simulink model "PMSM_FOC_MPC"  (R2024b)
settings: Solver=ode4  StartTime=0.0  StopTime=2  FixedStep=1e-6  RelTol=1e-3
InitFcn:
  | %% Motor Parameters
  | Rs = 0.9585;
  | Ls = 0.00525;
  | 
  | %% Observer Parameters
  | K = [817.42 0;
  |       0      817.42];
  | 
  | %% State Matrix
  | A = [ -Rs/Ls      0;
  |         0     -Rs/Ls ];
  | 
  | %% Input Matrix
  | B = [ 1/Ls      0;
  |         0     1/Ls ];
  | 
  | %% Output Matrix
  | C = [1 0;
  |      0 1];
  | 
  | %% Feedthrough
  | D = zeros(2,2);
values from neighbouring files (symbols this model uses):
  V = VPH - mean(VPH)    [three_level_inverter.m]
libraries: spsabctoAlphaBetaZeroLib x3, spsDCVoltageSourceLib x1, spsPermanentMagnetSynchronousMachineLib x1, spsThreePhaseVIMeasurementLib x1, spsUniversalBridgeLib x1, sps_lib x1, slpidlib x1
settings Model: SimulationMode=accelerator  Creator=killa  LastModifiedBy=killa

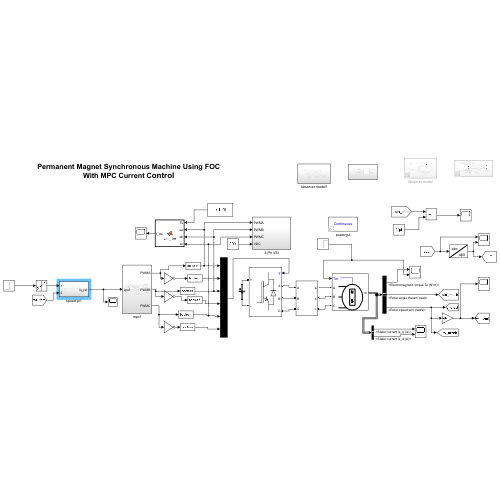
[thumbnail: Simulink's stored preview of the top-level diagram]
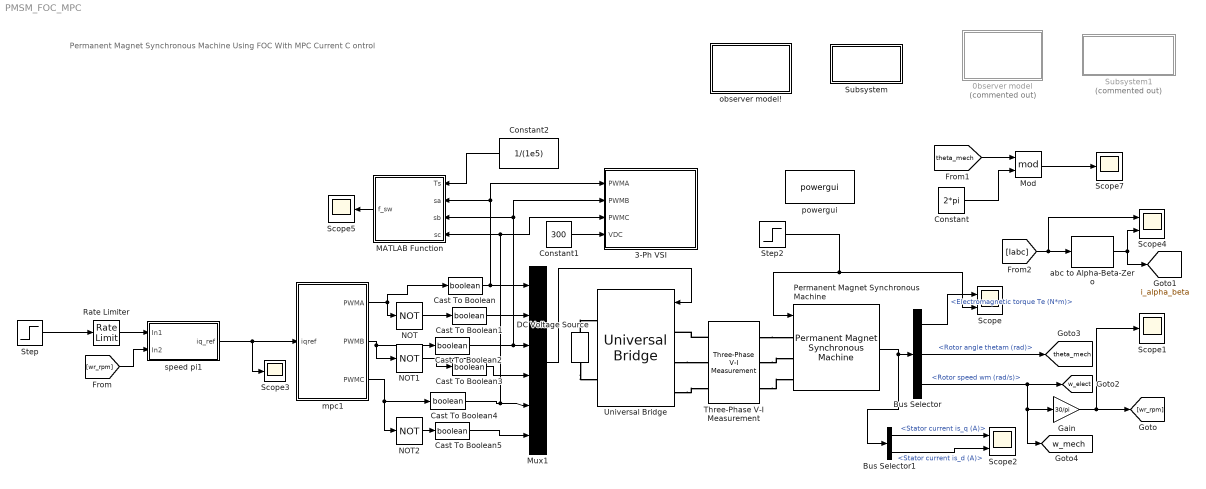
== system PMSM_FOC_MPC ==
  note: Permanent Magnet Synchronous Machine Using FOC With MPC Current C ontrol
  0bserver model : Subsystem  Commented=on
  3-Ph VSI : Subsystem
  Bus Selector : BusSelector  OutputSignals=Electromagnetic torque Te (N*m),Rotor angle thetam (rad),Rotor speed wm (rad/s)
  Bus Selector1 : BusSelector  OutputSignals=Stator current is_q (A),Stator current is_d (A)
  Cast To Boolean{,1..5} (6 alike) : DataTypeConversion  OutDataTypeStr=boolean  SaturateOnIntegerOverflow=off  RndMeth=Floor
  Constant : Constant  Value=2*pi
  Constant1 : Constant  Value=300
  Constant2 : Constant  Value=1/(1e5)
  DC Voltage Source : spsDCVoltageSourceLib/DC Voltage Source  Amplitude=300  Measurements=None
  Gain : Gain  Gain=30/pi
  MATLAB Function : MATLAB Function  TreatAsAtomicUnit=on
  Mod : Math  Operator=mod
  Mux1 : Mux  Inputs=6
  NOT : Logic  Operator=NOT  IconShape=distinctive  AllPortsSameDT=off  OutDataTypeStr=boolean
  NOT1 : Logic  Operator=NOT  IconShape=distinctive  AllPortsSameDT=off  OutDataTypeStr=boolean
  NOT2 : Logic  Operator=NOT  IconShape=distinctive  AllPortsSameDT=off  OutDataTypeStr=boolean
  Permanent Magnet Synchronous Machine : spsPermanentMagnetSynchronousMachineLib/Permanent Magnet Synchronous Machine  NbPhases=3  FluxDistribution=Sinusoidal  RotorType=Round  MechanicalLoad=Torque Tm  PresetModel="05:  8 Nm 300 Vdc 2000 RPM - 10 Nm"  ShowDetailedParameters=on  MeasurementBus=off  Resistance=0.9585  Inductance=8.5e-3  dqInductances=[8.5e-3,8.5e-3]  La=0.00525  MachineConstant=Flux linkage established by magnets (V.s)  Flux=0.1827  VoltageCst=132.5525  TorqueCst=1.0962  Flat=120  Mechanical=[0.0006329 0.0003035 4 0]  PolePairs=4  InitialConditions=[0,0, 0,0]  InitialConditions5ph=[0 0 0 0 0 0]  RefAngle=Aligned with phase A axis (original Park)  IterativeDiscreteModel=Trapezoidal non iterative  TsBlock=-1  TsPowergui=0
  Rate Limiter : RateLimiter  RisingSlewLimit=10000  FallingSlewLimit=-10000
  Scope : Scope  NumInputPorts=2
  Scope{1,3,5,7} (4 alike) : Scope
  Scope2 : Scope  NumInputPorts=2
  Scope4 : Scope  NumInputPorts=2
  Step : Step  Before=500  After=1500  SampleTime=0
  Step2 : Step  Time=0.5  Before=4  After=8  SampleTime=0
  Subsystem : Subsystem
  Subsystem1 : Subsystem  Commented=on
  Three-Phase V-I Measurement : spsThreePhaseVIMeasurementLib/Three-Phase V-I Measurement  VoltageMeasurement=no  SetLabelV=on  LabelV=Vabc  Vpu=off  VpuLL=off  CurrentMeasurement=yes  SetLabelI=on  LabelI=Iabc  Ipu=off  Pbase=100e6  Vbase=500e3  OutputType=Complex  PhasorSimulation=off  PSBequivalent=0
  Universal Bridge : spsUniversalBridgeLib/Universal Bridge  Arms=3  SnubberResistance=1e5  SnubberCapacitance=inf  Device=IGBT / Diodes  Ron=1e-3  Lon=0  ForwardVoltages="[  0  0  ]"  ForwardVoltage=0  GTOparameters=[ 10e-6 , 20e-6 ]  IGBTparameters=[ 1e-6 , 2e-6 ]  Measurements=None  Measurements_2=None  converterType=Rectifier
  abc to Alpha-Beta-Zero : spsabctoAlphaBetaZeroLib/abc to Alpha-Beta-Zero
  mpc1 : Subsystem
  observer model! : Subsystem
  powergui : sps_lib/powergui  Priority=1  SimulationMode=Continuous  SampleTime=50e-6  frequency=60  Iterations=50  frequencyindice=0  Pbase=100e6  ErrMax=1e-4  UnitsV=kV  UnitsW=MW  buscounter=0  FunctionMessages=off  echomessages=off  EnableUseOfTLC=off  CurrentSourceSwitches=off  DisableSnubberDevices=off  DisableRonSwitches=off  DisableVfSwitches=off  DisplayEquations=off  AutomaticDiscreteSolvers=off  SolverType=Tustin/Backward Euler (TBE)  Interpol=off  ExternalGateDelay=off  methode=off  Ts=100  x0status=blocks  SPID=on  SwTol=0  HookPort=off  NonlinearTolerance=1e-4  nMaxIteration=100  ContinueOnMaxIteration=off  RestoreLinks=warning  ResistiveCurrentMeasurement=off  Frange=[0:2:500]  Ylog=off  Xlog=on  ShowGrid=off  save=off  variable=ZData  structure=0  ZoomFFT=off  StartTime=0.0  cycles=1  DisplayStyle=1  fundamental=60  FreqAxis=off  MaxFrequency=1000  frequencyindicesteady=1  RmsSteady=1  display=off
  speed pi1 : Subsystem
  tag scope: i_alpha_beta=global, theta_mech=global, w_elect=global, w_mech=global
  wires:
  Permanent Magnet Synchronous Machine/1 -> Bus Selector1/1, Bus Selector/1
  Bus Selector/2 -> [theta_mech]  "<Rotor angle thetam (rad)>"
  Bus Selector/3 -> [w_mech], Gain/1, [w_elect]  "<Rotor speed wm (rad/s)>"
  Bus Selector/1 -> Scope/1  "<Electromagnetic torque Te (N*m)>"
  Gain/1 -> [wr_rpm], Scope1/1
  Cast To Boolean/1 -> Mux1/1, 3-Ph VSI/1(PWMA), MATLAB Function/2(sa)
  mpc1/1(PWMA) -> Cast To Boolean/1, NOT/1
  NOT/1 -> Cast To Boolean1/1
  Cast To Boolean1/1 -> Mux1/2
  mpc1/2(PWMB) -> Cast To Boolean2/1, NOT1/1
  NOT1/1 -> Cast To Boolean3/1
  mpc1/3(PWMC) -> Cast To Boolean4/1, NOT2/1
  NOT2/1 -> Cast To Boolean5/1
  Cast To Boolean2/1 -> 3-Ph VSI/2(PWMB), MATLAB Function/3(sb), Mux1/3
  Cast To Boolean3/1 -> Mux1/4
  Cast To Boolean4/1 -> 3-Ph VSI/3(PWMC), MATLAB Function/4(sc), Mux1/5
  Cast To Boolean5/1 -> Mux1/6
  Mux1/1 -> Universal Bridge/1
  [Iabc] -> abc to Alpha-Beta-Zero/1, Scope4/1
  Constant1/1 -> 3-Ph VSI/4(VDC)
  Step2/1 -> Scope/2, Permanent Magnet Synchronous Machine/1
  Bus Selector1/1 -> Scope2/1  "<Stator current is_q (A)>"
  Bus Selector1/2 -> Scope2/2  "<Stator current is_d (A)>"
  Constant2/1 -> MATLAB Function/1(Ts)
  MATLAB Function/1(f_sw) -> Scope5/1
  [wr_rpm] -> speed pi1/2(In2)
  speed pi1/1(iq_ref) -> mpc1/1(iqref), Scope3/1
  Step/1 -> Rate Limiter/1
  abc to Alpha-Beta-Zero/1 -> [i_alpha_beta], Scope4/2
  [theta_mech] -> Mod/1
  Constant/1 -> Mod/2
  Mod/1 -> Scope7/1
  Rate Limiter/1 -> speed pi1/1(In1)
  connections:
  DC Voltage Source/RConn1 -- Universal Bridge/RConn1
  DC Voltage Source/LConn1 -- Universal Bridge/RConn2
  Three-Phase V-I Measurement/LConn1 -- Universal Bridge/LConn1
  Universal Bridge/LConn2 -- Three-Phase V-I Measurement/LConn2
  Universal Bridge/LConn3 -- Three-Phase V-I Measurement/LConn3
  Three-Phase V-I Measurement/RConn1 -- Permanent Magnet Synchronous Machine/LConn1
  Three-Phase V-I Measurement/RConn2 -- Permanent Magnet Synchronous Machine/LConn2
  Three-Phase V-I Measurement/RConn3 -- Permanent Magnet Synchronous Machine/LConn3

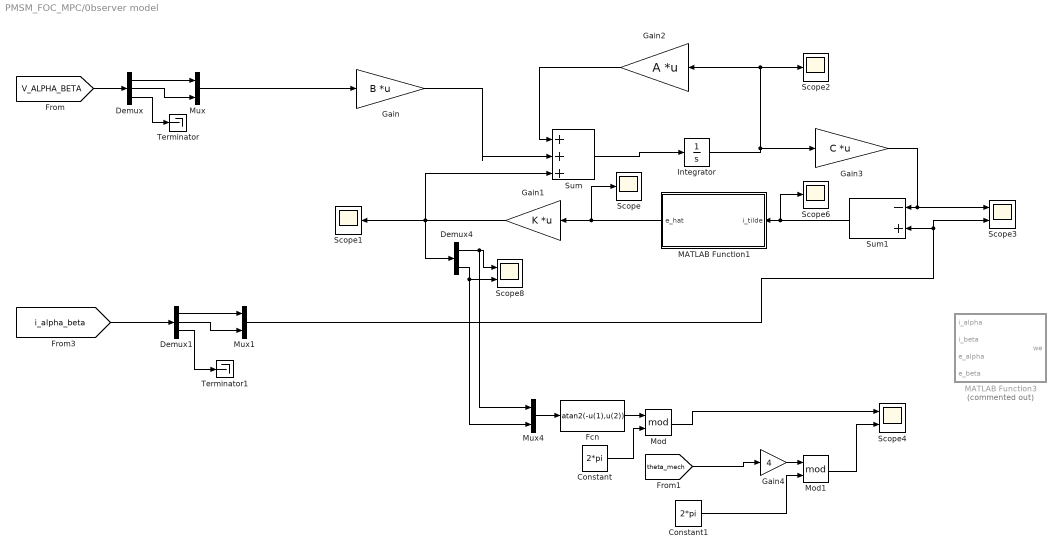
== system PMSM_FOC_MPC/0bserver model ==
  Constant : Constant  Value=2*pi
  Constant1 : Constant  Value=2*pi
  Demux : Demux  Outputs=3
  Demux1 : Demux  Outputs=3
  Demux4 : Demux  Outputs=2
  Fcn : Fcn  Expr=atan2(-u(1),u(2))
  Gain : Gain  Gain=B  Multiplication=Matrix(K*u)
  Gain1 : Gain  Gain=K  Multiplication=Matrix(K*u)
  Gain2 : Gain  Gain=A  Multiplication=Matrix(K*u)
  Gain3 : Gain  Gain=C  Multiplication=Matrix(K*u)
  Gain4 : Gain  Gain=4
  Integrator : Integrator
  MATLAB Function1 : MATLAB Function  TreatAsAtomicUnit=on
  MATLAB Function3 : MATLAB Function  Commented=on  TreatAsAtomicUnit=on
  Mod : Math  Operator=mod
  Mod1 : Math  Operator=mod
  Mux : Mux  Inputs=2
  Mux1 : Mux  Inputs=2
  Mux4 : Mux  Inputs=2
  Scope{,1..2,6} (4 alike) : Scope
  Scope3 : Scope  NumInputPorts=2
  Scope4 : Scope  NumInputPorts=2
  Scope8 : Scope  NumInputPorts=2
  Sum : Sum  Inputs=|+++
  Sum1 : Sum  Inputs=-+
  Terminator : Terminator
  Terminator1 : Terminator
  wires:
  Integrator/1 -> Scope2/1, Gain2/1, Gain3/1
  Gain2/1 -> Sum/1
  Fcn/1 -> Mod/1
  Sum/1 -> Integrator/1
  Constant/1 -> Mod/2
  Gain/1 -> Sum/2
  Mux4/1 -> Fcn/1
  Gain3/1 -> Scope3/1, Sum1/1
  [V_ALPHA_BETA] -> Demux/1
  Demux/1 -> Mux/1
  Demux/2 -> Mux/2
  Mux/1 -> Gain/1
  Demux/3 -> Terminator/1
  Demux1/1 -> Mux1/1
  Demux1/2 -> Mux1/2
  Demux1/3 -> Terminator1/1
  [i_alpha_beta] -> Demux1/1
  Mux1/1 -> Scope3/2, Sum1/2
  Sum1/1 -> Scope6/1, MATLAB Function1/1(i_tilde)
  MATLAB Function1/1(e_hat) -> Scope/1, Gain1/1
  Gain1/1 -> Demux4/1, Scope1/1, Sum/3
  Constant1/1 -> Mod1/2
  [theta_mech] -> Gain4/1
  Demux4/1 -> Mux4/1, Scope8/1
  Demux4/2 -> Mux4/2, Scope8/2
  Mod/1 -> Scope4/1
  Mod1/1 -> Scope4/2
  Gain4/1 -> Mod1/1

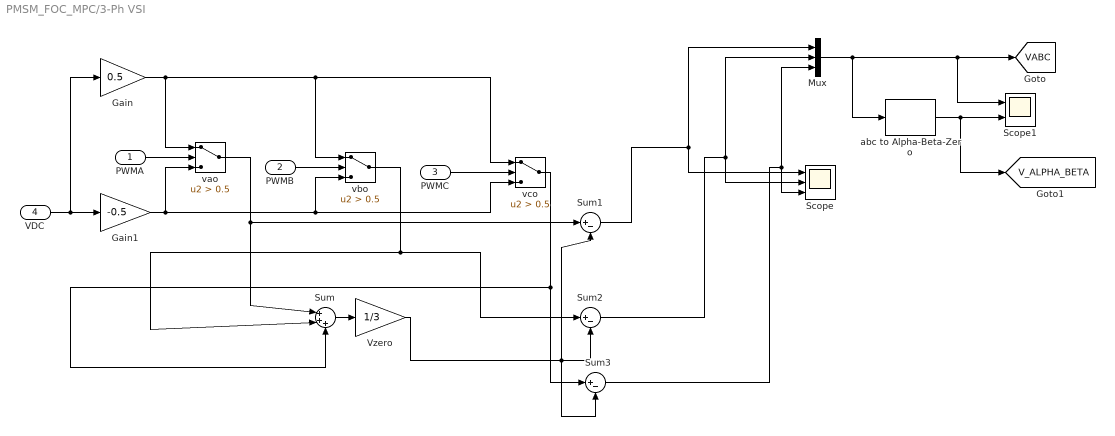
== system PMSM_FOC_MPC/3-Ph VSI ==
  PWMA : Inport
  PWMB : Inport  Port=2
  PWMC : Inport  Port=3
  VDC : Inport  Port=4
  Gain : Gain  Gain=0.5
  Gain1 : Gain  Gain=-0.5
  Mux : Mux  Inputs=3
  Scope : Scope  NumInputPorts=3
  Scope1 : Scope  NumInputPorts=2
  Sum : Sum  Inputs=|+++
  Sum1 : Sum  Inputs=|+-
  Sum2 : Sum  Inputs=|+-
  Sum3 : Sum  Inputs=|+-
  Vzero : Gain  Gain=1/3
  abc to Alpha-Beta-Zero : spsabctoAlphaBetaZeroLib/abc to Alpha-Beta-Zero
  vao : Switch  Criteria=u2 > Threshold  Threshold=0.5  SaturateOnIntegerOverflow=off  InputSameDT=off
  vbo : Switch  Criteria=u2 > Threshold  Threshold=0.5  SaturateOnIntegerOverflow=off  InputSameDT=off
  vco : Switch  Criteria=u2 > Threshold  Threshold=0.5  SaturateOnIntegerOverflow=off  InputSameDT=off
  tag scope: VABC=global, V_ALPHA_BETA=global
  wires:
  Gain/1 -> vao/1, vbo/1, vco/1
  Gain1/1 -> vao/3, vbo/3, vco/3
  VDC/1 -> Gain/1, Gain1/1
  PWMA/1 -> vao/2
  PWMB/1 -> vbo/2
  PWMC/1 -> vco/2
  vbo/1 -> Sum/2, Sum2/1
  vco/1 -> Sum/3, Sum3/1
  Sum/1 -> Vzero/1
  vao/1 -> Sum/1, Sum1/1
  Sum1/1 -> Mux/1, Scope/1
  Sum2/1 -> Mux/2, Scope/2
  Sum3/1 -> Mux/3, Scope/3
  Vzero/1 -> Sum3/2, Sum2/2, Sum1/2
  Mux/1 -> abc to Alpha-Beta-Zero/1, Scope1/1, [VABC]
  abc to Alpha-Beta-Zero/1 -> [V_ALPHA_BETA], Scope1/2

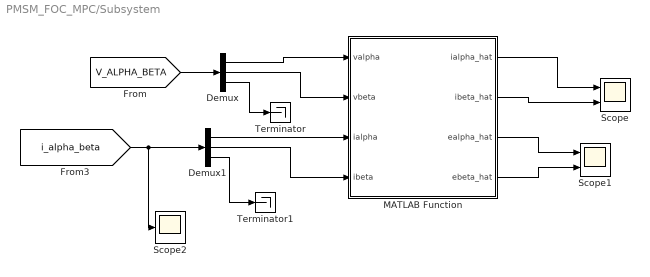
== system PMSM_FOC_MPC/Subsystem ==
  Demux : Demux  Outputs=3
  Demux1 : Demux  Outputs=3
  MATLAB Function : MATLAB Function  TreatAsAtomicUnit=on
  Scope : Scope  NumInputPorts=2
  Scope1 : Scope  NumInputPorts=2
  Scope2 : Scope
  Terminator : Terminator
  Terminator1 : Terminator
  wires:
  [i_alpha_beta] -> Scope2/1, Demux1/1
  Demux1/3 -> Terminator1/1
  Demux/3 -> Terminator/1
  [V_ALPHA_BETA] -> Demux/1
  Demux/1 -> MATLAB Function/1(valpha)
  Demux/2 -> MATLAB Function/2(vbeta)
  Demux1/1 -> MATLAB Function/3(ialpha)
  Demux1/2 -> MATLAB Function/4(ibeta)
  MATLAB Function/1(ialpha_hat) -> Scope/1
  MATLAB Function/2(ibeta_hat) -> Scope/2
  MATLAB Function/3(ealpha_hat) -> Scope1/1
  MATLAB Function/4(ebeta_hat) -> Scope1/2

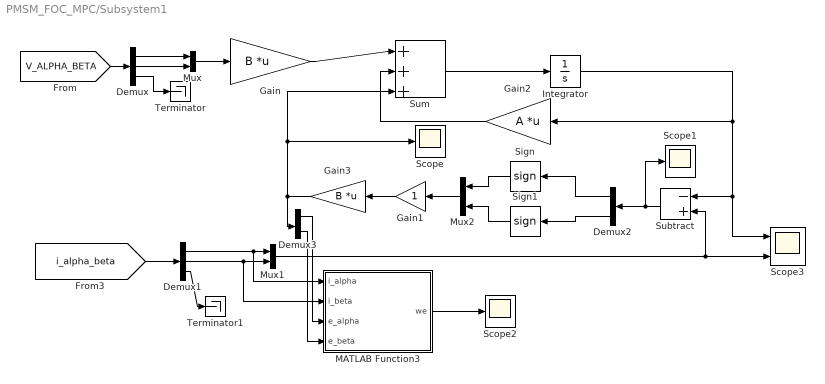
== system PMSM_FOC_MPC/Subsystem1 ==
  Demux : Demux  Outputs=3
  Demux1 : Demux  Outputs=3
  Demux2 : Demux  Outputs=2
  Demux3 : Demux  Outputs=2
  Gain : Gain  Gain=B  Multiplication=Matrix(K*u)
  Gain1 : Gain
  Gain2 : Gain  Gain=A  Multiplication=Matrix(K*u)
  Gain3 : Gain  Gain=B  Multiplication=Matrix(K*u)
  Integrator : Integrator
  MATLAB Function3 : MATLAB Function  TreatAsAtomicUnit=on
  Mux : Mux  Inputs=2
  Mux1 : Mux  Inputs=2
  Mux2 : Mux  Inputs=2
  Scope : Scope
  Scope1 : Scope
  Scope2 : Scope
  Scope3 : Scope  NumInputPorts=2
  Sign : Signum
  Sign1 : Signum
  Subtract : Sum  Inputs=-+
  Sum : Sum  Inputs=|+++
  Terminator : Terminator
  Terminator1 : Terminator
  wires:
  [i_alpha_beta] -> Demux1/1
  Demux1/3 -> Terminator1/1
  Demux1/2 -> MATLAB Function3/2(i_beta), Mux1/2
  Demux1/1 -> MATLAB Function3/1(i_alpha), Mux1/1
  Demux/3 -> Terminator/1
  Mux/1 -> Gain/1
  Demux/2 -> Mux/2
  Demux/1 -> Mux/1
  [V_ALPHA_BETA] -> Demux/1
  Sum/1 -> Integrator/1
  Integrator/1 -> Subtract/1, Scope3/1, Gain2/1
  Mux1/1 -> Subtract/2, Scope3/2
  Gain/1 -> Sum/1
  Gain2/1 -> Sum/2
  Demux2/1 -> Sign/1
  Demux2/2 -> Sign1/1
  Sign/1 -> Mux2/1
  Sign1/1 -> Mux2/2
  Mux2/1 -> Gain1/1
  Subtract/1 -> Scope1/1, Demux2/1
  Gain1/1 -> Gain3/1
  Gain3/1 -> Scope/1, Sum/3, Demux3/1
  Demux3/1 -> MATLAB Function3/3(e_alpha)
  Demux3/2 -> MATLAB Function3/4(e_beta)
  MATLAB Function3/1(we) -> Scope2/1

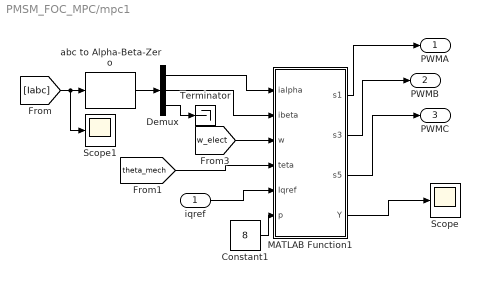
== system PMSM_FOC_MPC/mpc1 ==
  iqref : Inport
  Constant1 : Constant  Value=8
  Demux : Demux  Outputs=3
  MATLAB Function1 : MATLAB Function  TreatAsAtomicUnit=on
  Scope : Scope
  Scope1 : Scope
  Terminator : Terminator
  abc to Alpha-Beta-Zero : spsabctoAlphaBetaZeroLib/abc to Alpha-Beta-Zero
  PWMA : Outport
  PWMB : Outport  Port=2
  PWMC : Outport  Port=3
  wires:
  iqref/1 -> MATLAB Function1/5(Iqref)
  Constant1/1 -> MATLAB Function1/6(p)
  abc to Alpha-Beta-Zero/1 -> Demux/1
  Demux/1 -> MATLAB Function1/1(ialpha)
  Demux/2 -> MATLAB Function1/2(ibeta)
  Demux/3 -> Terminator/1
  [w_elect] -> MATLAB Function1/3(w)
  [theta_mech] -> MATLAB Function1/4(teta)
  [Iabc] -> Scope1/1, abc to Alpha-Beta-Zero/1
  MATLAB Function1/1(s1) -> PWMA/1
  MATLAB Function1/2(s3) -> PWMB/1
  MATLAB Function1/3(s5) -> PWMC/1
  MATLAB Function1/4(Y) -> Scope/1

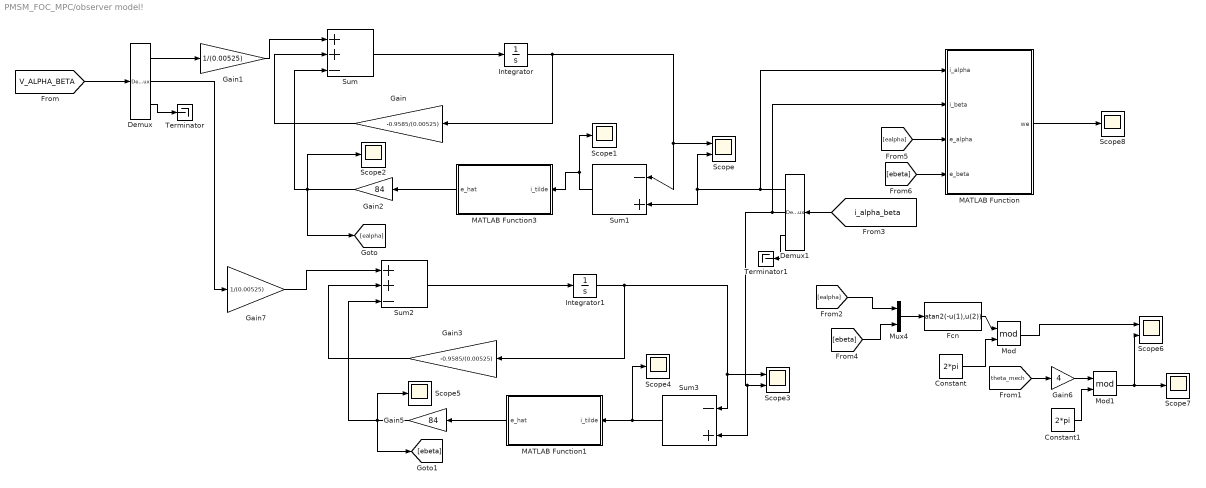
== system PMSM_FOC_MPC/observer model! ==
  Constant : Constant  Value=2*pi
  Constant1 : Constant  Value=2*pi
  Demux : Demux  Outputs=3
  Demux1 : Demux  Outputs=3
  Fcn : Fcn  Expr=atan2(-u(1),u(2))
  Gain : Gain  Gain=-0.9585/(0.00525)
  Gain1 : Gain  Gain=1/(0.00525)
  Gain2 : Gain  Gain=84
  Gain3 : Gain  Gain=-0.9585/(0.00525)
  Gain5 : Gain  Gain=84
  Gain6 : Gain  Gain=4
  Gain7 : Gain  Gain=1/(0.00525)
  Integrator : Integrator
  Integrator1 : Integrator
  MATLAB Function : MATLAB Function  TreatAsAtomicUnit=on
  MATLAB Function1 : MATLAB Function  TreatAsAtomicUnit=on
  MATLAB Function3 : MATLAB Function  TreatAsAtomicUnit=on
  Mod : Math  Operator=mod
  Mod1 : Math  Operator=mod
  Mux4 : Mux  Inputs=2
  Scope : Scope  NumInputPorts=2
  Scope{1..2,4..5,7..8} (6 alike) : Scope
  Scope3 : Scope  NumInputPorts=2
  Scope6 : Scope  NumInputPorts=2
  Sum : Sum  Inputs=|++-
  Sum1 : Sum  Inputs=|-+
  Sum2 : Sum  Inputs=|++-
  Sum3 : Sum  Inputs=|-+
  Terminator : Terminator
  Terminator1 : Terminator
  wires:
  [V_ALPHA_BETA] -> Demux/1
  Demux/3 -> Terminator/1
  Demux/1 -> Gain1/1
  Sum/1 -> Integrator/1
  Gain/1 -> Sum/2
  Sum1/1 -> MATLAB Function3/1(i_tilde), Scope1/1
  Gain2/1 -> [ealpha], Sum/3, Scope2/1
  Demux/2 -> Gain7/1
  Gain3/1 -> Sum2/2
  Sum3/1 -> Scope4/1, MATLAB Function1/1(i_tilde)
  Sum2/1 -> Integrator1/1
  Gain5/1 -> Sum2/3, [ebeta], Scope5/1
  [theta_mech] -> Gain6/1
  Mux4/1 -> Fcn/1
  Constant1/1 -> Mod1/2
  Constant/1 -> Mod/2
  Mod1/1 -> Scope6/2, Scope7/1
  Fcn/1 -> Mod/1
  Mod/1 -> Scope6/1
  [ealpha] -> Mux4/1
  [ebeta] -> Mux4/2
  Gain6/1 -> Mod1/1
  Integrator/1 -> Gain/1, Sum1/1, Scope/1
  Integrator1/1 -> Gain3/1, Sum3/1, Scope3/1
  Gain1/1 -> Sum/1
  Gain7/1 -> Sum2/1
  MATLAB Function3/1(e_hat) -> Gain2/1
  MATLAB Function1/1(e_hat) -> Gain5/1
  [i_alpha_beta] -> Demux1/1
  Demux1/3 -> Terminator1/1
  Demux1/1 -> MATLAB Function/1(i_alpha), Sum1/2, Scope/2
  Demux1/2 -> MATLAB Function/2(i_beta), Sum3/2, Scope3/2
  [ealpha] -> MATLAB Function/3(e_alpha)
  [ebeta] -> MATLAB Function/4(e_beta)
  MATLAB Function/1(we) -> Scope8/1

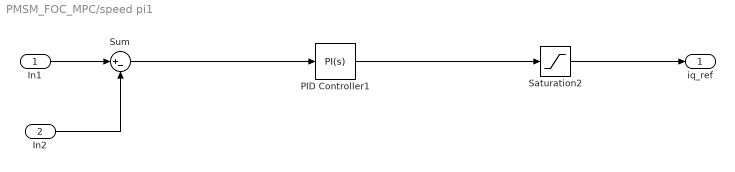
== system PMSM_FOC_MPC/speed pi1 ==
  In1 : Inport
  In2 : Inport  Port=2
  PID Controller1 : slpidlib/PID Controller  Controller=PI  Form=Parallel  TimeDomain=Continuous-time  UseExternalTs=off  SampleTime=-1  IntegratorMethod=Forward Euler  FilterMethod=Forward Euler  ControllerParametersSource=internal  P=0.5  I=5  UseKiTs=off  D=0  UseExternalDerivativeSource=off  N=100  UseFilter=on  TunerSelectOption=Transfer Function Based (PID Tuner App)  InitialConditionSource=internal  InitialConditionForIntegrator=0  InitialConditionForFilter=0  DifferentiatorICPrevScaledInput=0  ExternalReset=none  TrackingMode=off  Kt=1  LimitOutput=on  SatLimitsSource=internal  UpperSaturationLimit=inf  LowerSaturationLimit=-inf  LinearizeAsGain=on  AntiWindupMode=clamping  Kb=5/0.5  LimitIntegrator=off  UpperIntegratorSaturationLimit=inf  LowerIntegratorSaturationLimit=-inf  POutMin=[]  POutMax=[]  IOutMin=[]  IOutMax=[]  DOutMin=[]  DOutMax=[]  NOutMin=[]  NOutMax=[]  SumOutMin=[]  SumOutMax=[]  SaturationOutMin=[]  SaturationOutMax=[]  PParamMin=[]  PParamMax=[]  IParamMin=[]  IParamMax=[]  DParamMin=[]  DParamMax=[]  NParamMin=[]  NParamMax=[]  KbParamMin=[]  KbParamMax=[]  KtParamMin=[]  KtParamMax=[]  KbOutMin=[]  KbOutMax=[]  KtOutMin=[]  KtOutMax=[]  IntegratorOutMin=[]  IntegratorOutMax=[]  FilterOutMin=[]  FilterOutMax=[]  SumI1OutMin=[]  SumI1OutMax=[]  SumI2OutMin=[]  SumI2OutMax=[]  SumI3OutMin=[]  SumI3OutMax=[]  SumI4OutMin=[]  SumI4OutMax=[]  SumDOutMin=[]  SumDOutMax=[]  DifferentiatorOutMin=[]  DifferentiatorOutMax=[]  FilterDiffOutCoefMin=[]  FilterDiffOutCoefMax=[]  ReciprocalOutMin=[]  ReciprocalOutMax=[]  SumDenOutMin=[]  SumDenOutMax=[]  SumNumOutMin=[]  SumNumOutMax=[]  DivideOutMin=[]  DivideOutMax=[]  UdiffTsProdOutMin=[]  UdiffTsProdOutMax=[]  NTsProdOutMin=[]  NTsProdOutMax=[]  UintegralTsProdOutMin=[]  UintegralTsProdOutMax=[]  UngainTsProdOutMin=[]  UngainTsProdOutMax=[]  ClampingZeroOutDataTypeStr=Inherit: Inherit via back propagation  ClampingZeroOutMin=[]  ClampingZeroOutMax=[]  FilterDenConstantOutDataTypeStr=Inherit: Inherit via back propagation  FilterDenConstantOutMin=[]  FilterDenConstantOutMax=[]  PCopyOutDataTypeStr=Inherit: Inherit via back propagation  PCopyOutMin=[]  PCopyOutMax=[]  NCopyOutDataTypeStr=Inherit: Inherit via back propagation  NCopyOutMin=[]  NCopyOutMax=[]  IntegratorContinuousStateAttributes=''  IntegratorStateMustResolveToSignalObject=off  IntegratorRTWStateStorageClass=Auto  FilterContinuousStateAttributes=''  FilterStateMustResolveToSignalObject=off  FilterRTWStateStorageClass=Auto  ParallelPVariant=InternalParameters  IdealPVariant=Disabled  IVariant=InternalParameters  DVariant=Disabled  IntegratorVariant=Continuous  SatVariant=Enabled  AWVariant=ContClampingParallel  PCopyVariant=Disabled  TRVariant=Disabled  FdbkBlocksVariant=Forward  IdealPFdbkVariant=Disabled  SatFdbkVariant=Disabled  DerivativeFilterVariant=Disabled  NVariant=Disabled  NCopyVariant=Disabled_SignalSpec  FilterICVariant=Disabled  IntegratorICVariant=InternalICs  ExternalResetVariant=Disabled  TRSumVariant=Passthrough  SumFdbkVariant=Disabled  SumVariant=Sum_PI  TsampFilterVariant=InternalTs  TsampNgainVariant=Passthrough  TsampIntegralVariant=Disabled_SignalSpec  ExternalSaturationOutDataTypeStr=Inherit: Same as second input  DerivativeSourceVariant=Disabled  PreIntVariant=InternalPreInt
  Saturation2 : Saturate  UpperLimit=10  LowerLimit=-10
  Sum : Sum  Inputs=|+-
  iq_ref : Outport
  wires:
  In2/1 -> Sum/2
  In1/1 -> Sum/1
  PID Controller1/1 -> Saturation2/1
  Sum/1 -> PID Controller1/1
  Saturation2/1 -> iq_ref/1

== matlab function PMSM_FOC_MPC/MATLAB Function ==
  data: Ts input; f_sw output; sa input; sb input; sc input
function f_sw = calc_fsw(Ts,sa, sb, sc)
    persistent old_states total_transitions sample_count
   
    
    if isempty(old_states)
        old_states = [0 0 0];
        total_transitions = 0;
        sample_count = 0;
    end
   
   
    current_states = [sa, sb, sc];
   
   
    transitions = sum(abs(current_states - old_states));
   
       total_transitions = total_transitions + transitions;
    sample_count = sample_count + 1;
   

    old_states = double(current_states);
   
      if sample_count > 0
        f_sw = total_transitions / (2 * 3 * (sample_count * Ts));
    else
        f_sw = 0;
    end
end

== matlab function PMSM_FOC_MPC/observer model!/MATLAB Function1 ==
  data: i_tilde input; e_hat output
function e_hat = fcn(i_tilde)
%#codegen
%
% Input:
%   i_tilde : 2x1 current error vector
%             i_tilde = [i_alpha_tilde;
%                        i_beta_tilde]
%
% Output:
%   e_hat : 2x1 estimated back-EMF vector
%           e_hat = [e_alpha_hat;
%                    e_beta_hat]

%% Observer Parameters      % Observer gain
a  = 1;    % Smoothing parameter
n  = 1;        % Nonlinearity exponent

%% Soft-Sign Function
e_hat = ( i_tilde / (a + abs(i_tilde)^n) );

end

== matlab function PMSM_FOC_MPC/mpc1/MATLAB Function1 ==
  settings: updateMethod=DISCRETE
  data: ialpha input; s1 output; ibeta input; w input; teta input; Iqref input; p input; s3 output; s5 output; Y output
function [s1,s3,s5,Y] = fcn(ialpha,ibeta, w, teta, Iqref, p)

Vdc = 300;
fs = 1e5;
Ts = 1/fs;

Rs = 0.9585;
Ld = 0.00525;
Lq = 0.00525;
states = [0 0 0;1 0 0;1 1 0;0 1 0;0 1 1;0 0 1;1 0 1;1 1 1];
persistent x_opt
if isempty (x_opt)
    x_opt=1;
end
%imax = 10;
fluxlinkage = 0.1827;

% electrical angle and speed
tetaelec = (p/2)*teta;
welec = (p/2)*w;


% Park transform
Id = cos(tetaelec)*ialpha + sin(tetaelec)*ibeta;
Iq = -sin(tetaelec)*ialpha + cos(tetaelec)*ibeta;

% inverter voltage vectors
v0 = 0;

v1 = (2/3)*Vdc;

v2 = (1/3)*Vdc + 1j*(sqrt(3)/3)*Vdc;

v3 = (-1/3)*Vdc + 1j*(sqrt(3)/3)*Vdc;

v4 = (-2/3)*Vdc;

v5 = (-1/3)*Vdc - 1j*(sqrt(3)/3)*Vdc;

v6 = (1/3)*Vdc - 1j*(sqrt(3)/3)*Vdc;

v7 = 0;

vd = [v0 v1 v2 v3 v4 v5 v6 v7];

% optimization initialization
g_opt = 1e10;
x_opt = 1;

for i = 1:8
    
    % convert voltage vector to dq frame
    Vd = cos(tetaelec)*real(vd(i)) + sin(tetaelec)*imag(vd(i));
    
    Vq = -sin(tetaelec)*real(vd(i)) + cos(tetaelec)*imag(vd(i));
    
    % predicted currents
    Idnew = (Ts*Vd/Ld) + (1 - (Rs*Ts/Ld))*Id  + (welec*Ts*Lq/Ld)*Iq;
      
    Iqnew = (Ts*Vq/Lq) + (1 - (Rs*Ts/Lq))*Iq - (welec*Ts*Ld/Lq)*Id - (welec*Ts/Lq)*fluxlinkage;

    % cost function
    g = (Idnew)^2 + (Iqref - Iqnew)^2;

    % select optimal vector
    if g < g_opt
        
        g_opt = g;
        x_opt = i;
        
    end
end
s1 = states(x_opt,1);
s3 = states(x_opt,2);
s5 = states(x_opt,3);
Y=x_opt;

== matlab function PMSM_FOC_MPC/Subsystem1/MATLAB Function3 ==
  data: i_alpha input; i_beta input; e_alpha input; we output; e_beta input
function we = fcn(i_alpha,i_beta,e_alpha,e_beta)
%#codegen
%
% Inputs:
% e_alpha : Estimated alpha-axis back EMF
% e_beta  : Estimated beta-axis back EMF
% i_alpha : Alpha-axis current
% i_beta  : Beta-axis current
% psi     : Permanent magnet flux linkage (Wb)
%
% Output:
% we      : Electrical speed (rad/s)
psi = 0.1857;
% Avoid division by zero
eps = 1e-8;

% Numerator
num = (e_beta*i_alpha - e_alpha*i_beta);

% Denominator
den = psi*sqrt(i_alpha^2 + i_beta^2);

if den < eps
    we = 0;
else
    we = num/den;
end

end

== matlab function PMSM_FOC_MPC/0bserver model/MATLAB Function1 ==
  data: i_tilde input; e_hat output
function e_hat = fcn(i_tilde)
%#codegen
%
% Input:
%   i_tilde : 2x1 current error vector
%             i_tilde = [i_alpha_tilde;
%                        i_beta_tilde]
%
% Output:
%   e_hat : 2x1 estimated back-EMF vector
%           e_hat = [e_alpha_hat;
%                    e_beta_hat]

%% Observer Parameters      % Observer gain
a  = 0.1;    % Smoothing parameter
n  = 1;        % Nonlinearity exponent

%% Soft-Sign Function
e_hat = ( i_tilde ./ (a + abs(i_tilde).^n) );

end

== matlab function PMSM_FOC_MPC/0bserver model/MATLAB Function3 ==
  data: i_alpha input; i_beta input; e_alpha input; we output; e_beta input
function we = fcn(i_alpha,i_beta,e_alpha,e_beta)
%#codegen
%
% Inputs:
% e_alpha : Estimated alpha-axis back EMF
% e_beta  : Estimated beta-axis back EMF
% i_alpha : Alpha-axis current
% i_beta  : Beta-axis current
% psi     : Permanent magnet flux linkage (Wb)
%
% Output:
% we      : Electrical speed (rad/s)
psi = 0.1857;
% Avoid division by zero
eps = 1e-8;

% Numerator
num = (e_beta*i_alpha - e_alpha*i_beta);

% Denominator
den = psi*sqrt(i_alpha^2 + i_beta^2);

if den < eps
    we = 0;
else
    we = num/den;
end

end

== matlab function PMSM_FOC_MPC/observer model!/MATLAB Function ==
  data: i_alpha input; we output; i_beta input; e_alpha input; e_beta input
function we = fcn(i_alpha,i_beta,e_alpha,e_beta)
%#codegen
%
% Inputs:
% e_alpha : Estimated alpha-axis back EMF
% e_beta  : Estimated beta-axis back EMF
% i_alpha : Alpha-axis current
% i_beta  : Beta-axis current
% psi     : Permanent magnet flux linkage (Wb)
%
% Output:
% we      : Electrical speed (rad/s)
psi = 0.1857;
% Avoid division by zero
eps = 1e-8;

% Numerator
num = (e_beta*i_alpha - e_alpha*i_beta);

% Denominator
den = psi*sqrt(i_alpha^2 + i_beta^2);

if den < eps
    we = 0;
else
    we = num/den;
end

end

== matlab function PMSM_FOC_MPC/observer model!/MATLAB Function3 ==
  data: i_tilde input; e_hat output
function e_hat = fcn(i_tilde)
%#codegen
%
% Input:
%   i_tilde : 2x1 current error vector
%             i_tilde = [i_alpha_tilde;
%                        i_beta_tilde]
%
% Output:
%   e_hat : 2x1 estimated back-EMF vector
%           e_hat = [e_alpha_hat;
%                    e_beta_hat]

%% Observer Parameters      % Observer gain
a  = 1;    % Smoothing parameter
n  = 1;        % Nonlinearity exponent

%% Soft-Sign Function
e_hat = ( i_tilde / (a + abs(i_tilde)^n) );

end

== matlab function PMSM_FOC_MPC/Subsystem/MATLAB Function ==
  settings: updateMethod=DISCRETE
  data: valpha input; ialpha_hat output; vbeta input; ialpha input; ibeta input; ibeta_hat output; ealpha_hat output; ebeta_hat output
function [ialpha_hat, ibeta_hat, ealpha_hat, ebeta_hat] = ...
    PMSM_SMO(valpha, vbeta, ialpha, ibeta)

% =========================================================
% PMSM SENSORLESS SLIDING MODE OBSERVER
% Two states:
%       x1 = i_alpha
%       x2 = i_beta
%
% Inputs:
%       valpha, vbeta
%       ialpha, ibeta
%
% Outputs:
%       ialpha_hat, ibeta_hat
%       ealpha_hat, ebeta_hat
% =========================================================

% Motor parameters
Rs = 0.9585;
Ls = 0.00525;

% Sampling time
Ts = 1e-5;          % Change to your actual SMO sample time

% Sliding-mode parameters
Ks = 74;            % Sliding gain
phi = 0.01;         % Boundary layer

% Motor coefficients
A = Rs/Ls;
B = 1/Ls;

% =========================================================
% Observer states
% =========================================================
persistent ia_hat ib_hat

if isempty(ia_hat)
    ia_hat = 0;
    ib_hat = 0;
end

% =========================================================
% Current estimation error
% =========================================================
s_alpha = ialpha - ia_hat;
s_beta  = ibeta  - ib_hat;

% =========================================================
% Saturation function
% =========================================================
if abs(s_alpha) > phi
    sat_alpha = sign(s_alpha);
else
    sat_alpha = s_alpha/phi;
end

if abs(s_beta) > phi
    sat_beta = sign(s_beta);
else
    sat_beta = s_beta/phi;
end

% =========================================================
% Sliding-mode injection
% =========================================================
z_alpha = Ks * sat_alpha;
z_beta  = Ks * sat_beta;

% =========================================================
% Current observer
% =========================================================
d_ia_hat = -A*ia_hat + B*valpha + z_alpha;

d_ib_hat = -A*ib_hat + B*vbeta + z_beta;

% =========================================================
% Euler integration
% =========================================================
ia_hat = ia_hat + Ts*d_ia_hat;
ib_hat = ib_hat + Ts*d_ib_hat;

% =========================================================
% Back-EMF estimation
% =========================================================
% z = -Ls*e at sliding condition
%
% Therefore:
% e_hat = -z/Ls
% =========================================================

ealpha_hat = -z_alpha/Ls;
ebeta_hat  = -z_beta/Ls;

% =========================================================
% Outputs
% =========================================================
ialpha_hat = ia_hat;
ibeta_hat  = ib_hat;
